simulink model "Longitidunal_Vehicle_Dynamics"  (R2019b)
settings: Solver=VariableStepAuto  StartTime=0.0  StopTime=200  RelTol=1e-3
undefined symbols (not defined in the file): A, a1, a2, cx, g, h, J_w, l, m, mu0, mu1, r, ro, rw, v0
libraries: simulink x1
settings Model: Creator=xps  LastModifiedBy=yanbing_wang
settings SolverCC: ZeroCrossAlgorithm=Adaptive
settings DataIOCC: ReturnWorkspaceOutputs=off
settings DebuggingCC: MaxConsecutiveZCsMsg=none  MaskedZcDiagnostic=none  IgnoredZcDiagnostic=none  ArithmeticOperatorsInVariantConditions=warning
settings SFSimCC: SimUseLocalCustomCode=off  CustomCodeUndefinedFunction=UseInterfaceOnly
settings RTWCC: RTWUseLocalCustomCode=off
settings CodeAppCC: StateflowObjectComments=on

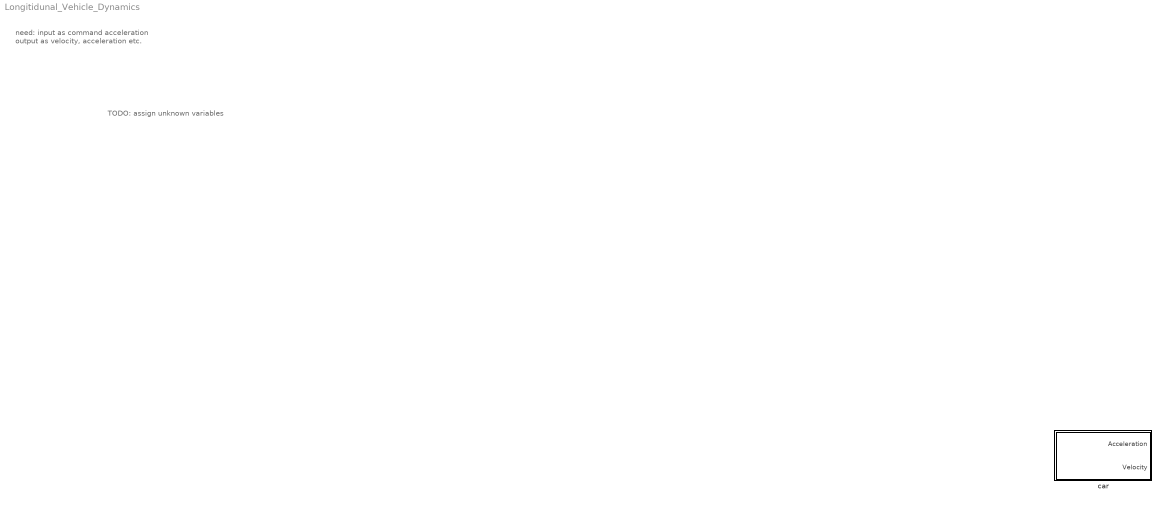
== system Longitidunal_Vehicle_Dynamics ==
  note: TODO: assign unknown variables
  note: need: input as command acceleration
      | output as velocity, acceleration etc.
  car : Subsystem

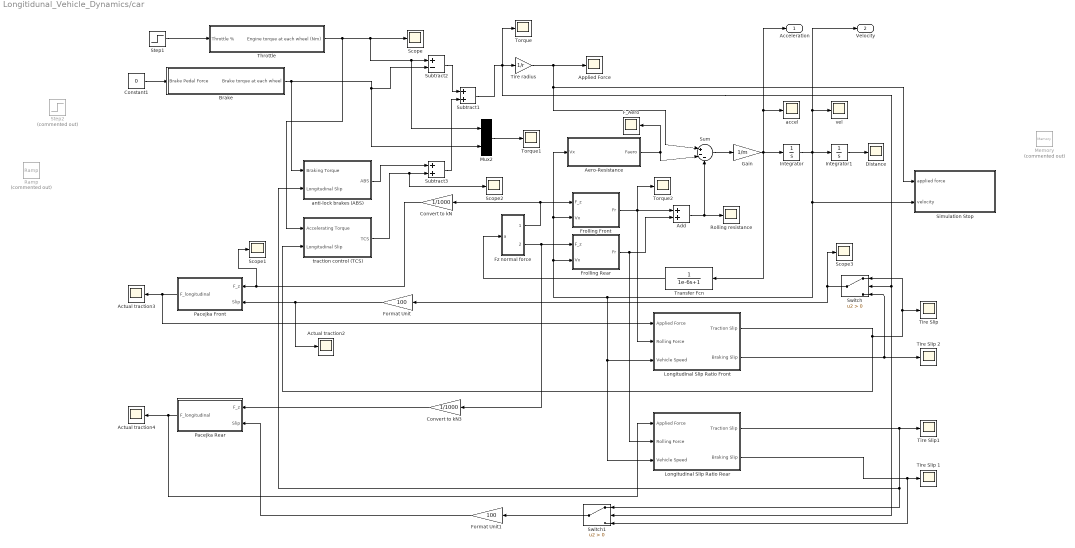
== system Longitidunal_Vehicle_Dynamics/car ==
  Actual traction2 : Scope
  Actual traction3 : Scope
  Actual traction4 : Scope
  Add : Sum
  Aero-Resistance : Subsystem
  Applied Force : Scope
  Brake : Subsystem
  Constant1 : Constant  Value=0
  Convert to kN : Gain  Gain=1/1000
  Convert to kN3 : Gain  Gain=1/1000
  Distance : Scope
  F_Aero : Scope
  Format Unit : Gain  Gain=100
  Format Unit1 : Gain  Gain=100
  Frolling Front : Subsystem
  Frolling Rear : Subsystem
  Fz normal force : Subsystem
  Gain : Gain  Gain=1/m
  Integrator : Integrator  InitialCondition=v0
  Integrator1 : Integrator
  Longitudinal Slip Ratio Front : Subsystem
  Longitudinal Slip Ratio Rear : Subsystem
  Memory : Memory  Commented=on
  Mux2 : Mux  Inputs=2
  Pacejka Front : Subsystem
  Pacejka Rear : Subsystem
  Ramp : simulink/Sources/Ramp  Commented=on  slope=1  start=50  InitialOutput=0
  "Rolling resistance " : Scope
  Scope{,1..3} (4 alike) : Scope
  Simulation Stop : Subsystem
  Step1 : Step  Time=100  After=50  SampleTime=50
  Step2 : Step  Commented=on  Time=100  After=50  SampleTime=1
  Subtract1 : Sum
  Subtract2 : Sum  Inputs=+-
  Subtract3 : Sum
  Sum : Sum  Inputs=|+--
  Switch : Switch  Criteria=u2 > Threshold
  Switch1 : Switch  Criteria=u2 > Threshold
  Throttle : Subsystem
  Tire Slip : Scope
  Tire Slip 1 : Scope
  Tire Slip 2 : Scope
  Tire Slip1 : Scope
  Tire radius : Gain  Gain=1/r
  Torque : Scope
  Torque1 : Scope
  Torque2 : Scope
  Transfer Fcn : TransferFcn  Denominator=[1e-6 1]
  accel : Scope
  anti-lock brakes (ABS) : Subsystem
  traction control (TCS) : Subsystem
  vel : Scope
  Acceleration : Outport
  Velocity : Outport  Port=2
  wires:
  Sum/1 -> Gain/1
  Pacejka Rear/1(F_longitudinal) -> Longitudinal Slip Ratio Rear/1(Applied Force), Actual traction4/1
  Step1/1 -> Throttle/1(Throttle %)
  Format Unit1/1 -> Pacejka Rear/2(Slip)
  Longitudinal Slip Ratio Rear/2(Braking Slip) -> Switch1/3, Tire Slip 1/1
  Integrator1/1 -> Distance/1
  Fz normal force/2(F_z2) -> Convert to kN3/1, Frolling Rear/1(F_z)
  Brake/1(Brake torque at each wheel) -> Subtract2/2, Mux2/2, anti-lock brakes (ABS)/1(Braking Torque)
  Longitudinal Slip Ratio Front/1(Traction Slip) -> traction control (TCS)/2(Longitudinal Slip), Switch/1, Tire Slip/1
  Frolling Rear/1(Fr) -> Longitudinal Slip Ratio Rear/2(Rolling Force), Add/2
  Aero-Resistance/1(Faero) -> Sum/2, F_Aero/1
  Subtract1/1 -> Torque/1, Switch/2, Switch1/2, Tire radius/1
  Subtract2/1 -> Subtract1/1
  Pacejka Front/1(F_longitudinal) -> Actual traction3/1, Longitudinal Slip Ratio Front/1(Applied Force)
  Mux2/1 -> Torque1/1
  traction control (TCS)/1(TCS) -> Scope2/1, Subtract3/2
  Longitudinal Slip Ratio Front/2(Braking Slip) -> Switch/3, Tire Slip 2/1
  Constant1/1 -> Brake/1(Brake Pedal Force)
  Tire radius/1 -> Simulation Stop/1(applied force), Sum/1, Applied Force/1
  Frolling Front/1(Fr) -> Longitudinal Slip Ratio Front/2(Rolling Force), Add/1, Torque2/1
  Longitudinal Slip Ratio Rear/1(Traction Slip) -> anti-lock brakes (ABS)/2(Longitudinal Slip), Switch1/1, Tire Slip1/1
  Subtract3/1 -> Subtract1/2
  anti-lock brakes (ABS)/1(ABS) -> Subtract3/1
  Switch/1 -> Format Unit/1, Scope3/1
  Convert to kN3/1 -> Pacejka Rear/1(F_z)
  Convert to kN/1 -> Scope1/1, Pacejka Front/1(F_z)
  Fz normal force/1(F_z1) -> Convert to kN/1, Frolling Front/1(F_z)
  Switch1/1 -> Format Unit1/1
  Integrator/1 -> Longitudinal Slip Ratio Rear/3(Vehicle Speed), Longitudinal Slip Ratio Front/3(Vehicle Speed), Frolling Front/2(Vx), Aero-Resistance/1(Vx), Frolling Rear/2(Vx), Simulation Stop/2(velocity), Velocity/1, vel/1, Integrator1/1
  Throttle/1(Engine torque at each wheel (Nm)) -> Scope/1, Subtract2/1, Mux2/1, traction control (TCS)/1(Accelerating Torque)
  Add/1 -> Sum/3, "Rolling resistance "/1
  Format Unit/1 -> Pacejka Front/2(Slip), Actual traction2/1
  Gain/1 -> Transfer Fcn/1, Acceleration/1, accel/1, Integrator/1
  Transfer Fcn/1 -> Fz normal force/1(a)

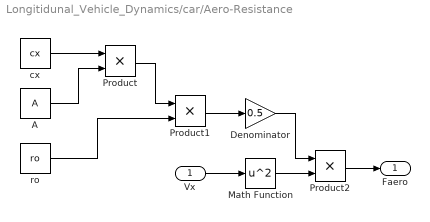
== system Longitidunal_Vehicle_Dynamics/car/Aero-Resistance ==
  Vx : Inport
  A : Constant  Value=A
  Denominator : Gain  Gain=0.5
  Math Function : Math  Operator=square  SaturateOnIntegerOverflow=on
  Product : Product
  Product1 : Product
  Product2 : Product
  cx : Constant  Value=cx
  ro : Constant  Value=ro
  Faero : Outport  VectorParamsAs1DForOutWhenUnconnected=off
  wires:
  A/1 -> Product/2
  Product1/1 -> Denominator/1
  Denominator/1 -> Product2/1
  Vx/1 -> Math Function/1
  Product2/1 -> Faero/1
  ro/1 -> Product1/2
  cx/1 -> Product/1
  Math Function/1 -> Product2/2
  Product/1 -> Product1/1

== system Longitidunal_Vehicle_Dynamics/car/Brake ==
  Brake Pedal Force : Inport
  Gain : Gain  Gain=400
  Gain1 : Gain
  r_static : Gain  Gain=0.3
  Brake torque at each wheel : Outport  VectorParamsAs1DForOutWhenUnconnected=off
  wires:
  Gain1/1 -> r_static/1
  Gain/1 -> Gain1/1
  Brake Pedal Force/1 -> Gain/1
  r_static/1 -> Brake torque at each wheel/1

== system Longitidunal_Vehicle_Dynamics/car/Frolling Front ==
  F_z : Inport
  Vx : Inport  Port=2
  Add : Sum
  Math Function : Math  Operator=square  SaturateOnIntegerOverflow=on
  Product : Product
  Product1 : Product
  mu0 : Constant  Value=mu0
  mu1 : Constant  Value=mu1
  Fr : Outport  VectorParamsAs1DForOutWhenUnconnected=off
  wires:
  Add/1 -> Product1/2
  Math Function/1 -> Product/2
  Product/1 -> Add/2
  mu0/1 -> Add/1
  mu1/1 -> Product/1
  Vx/1 -> Math Function/1
  Product1/1 -> Fr/1
  F_z/1 -> Product1/1

== system Longitidunal_Vehicle_Dynamics/car/Frolling Rear ==
  F_z : Inport
  Vx : Inport  Port=2
  Add : Sum
  Math Function : Math  Operator=square  SaturateOnIntegerOverflow=on
  Product : Product
  Product1 : Product
  mu0 : Constant  Value=mu0
  mu1 : Constant  Value=mu1
  Fr : Outport  VectorParamsAs1DForOutWhenUnconnected=off
  wires:
  F_z/1 -> Product1/1
  Product1/1 -> Fr/1
  Vx/1 -> Math Function/1
  mu1/1 -> Product/1
  mu0/1 -> Add/1
  Product/1 -> Add/2
  Math Function/1 -> Product/2
  Add/1 -> Product1/2

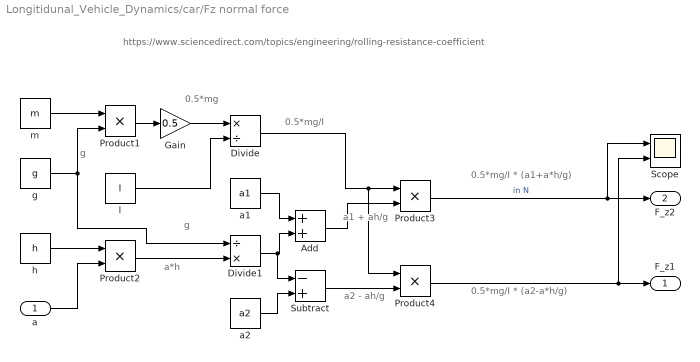
== system Longitidunal_Vehicle_Dynamics/car/Fz normal force ==
  note: https://www.sciencedirect.com/topics/engineering/rolling-resistance-coefficient
  note: a2 - ah/g
  note: a1 + ah/g
  note: 0.5*mg
  note: g
  note: a*h
  note: g
  note: 0.5*mg/I
  note: 0.5*mg/I * (a2-a*h/g)
  note: 0.5*mg/I * (a1+a*h/g)
  a : Inport
  Add : Sum
  Divide : Product  Inputs=*/
  Divide1 : Product  Inputs=/*
  Gain : Gain  Gain=0.5
  Product{1..4} (4 alike) : Product
  Scope : Scope  NumInputPorts=2
  Subtract : Sum  Inputs=-+
  a1 : Constant  Value=a1
  a2 : Constant  Value=a2
  g : Constant  Value=g
  h : Constant  Value=h
  l : Constant  Value=l
  m : Constant  Value=m
  F_z1 : Outport  VectorParamsAs1DForOutWhenUnconnected=off
  F_z2 : Outport  Port=2  VectorParamsAs1DForOutWhenUnconnected=off
  wires:
  m/1 -> Product1/1
  g/1 -> Divide1/1, Product1/2
  Product1/1 -> Gain/1
  Gain/1 -> Divide/1
  l/1 -> Divide/2
  h/1 -> Product2/1
  Product2/1 -> Divide1/2
  a1/1 -> Add/1
  Divide1/1 -> Subtract/1, Add/2
  Divide/1 -> Product4/1, Product3/1
  Add/1 -> Product3/2
  a2/1 -> Subtract/2
  Subtract/1 -> Product4/2
  Product4/1 -> Scope/2, F_z1/1
  Product3/1 -> Scope/1, F_z2/1  "in N"
  a/1 -> Product2/2

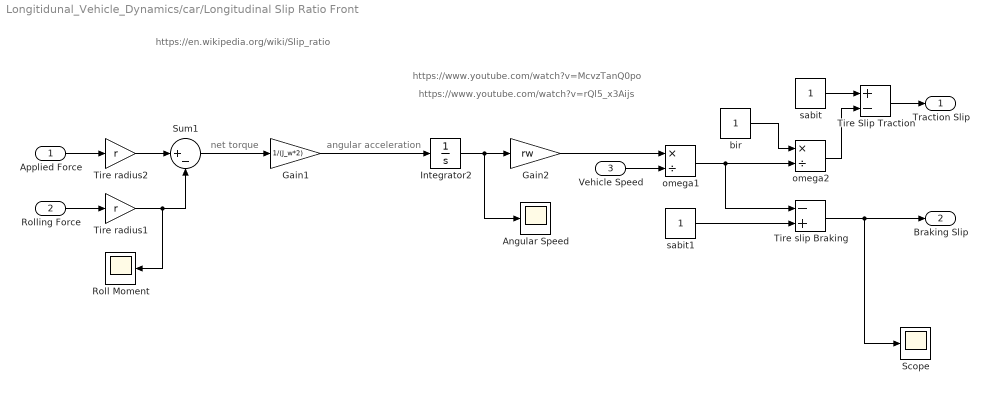
== system Longitidunal_Vehicle_Dynamics/car/Longitudinal Slip Ratio Front ==
  note: https://www.youtube.com/watch?v=McvzTanQ0po
  note: net torque
  note: https://www.youtube.com/watch?v=rQl5_x3Aijs
  note: angular acceleration
  note: https://en.wikipedia.org/wiki/Slip_ratio
  Applied Force : Inport
  Rolling Force : Inport  Port=2
  Vehicle Speed : Inport  Port=3
  Angular Speed : Scope
  Gain1 : Gain  Gain=1/(J_w*2)
  Gain2 : Gain  Gain=rw
  Integrator2 : Integrator  InitialCondition=0.00001
  Roll Moment : Scope
  Scope : Scope
  Sum1 : Sum  Inputs=|+-
  Tire Slip Traction : Sum  Inputs=+-
  Tire radius1 : Gain  Gain=r
  Tire radius2 : Gain  Gain=r
  Tire slip Braking : Sum  Inputs=-+
  bir : Constant
  omega1 : Product  Inputs=*/
  omega2 : Product  Inputs=*/
  sabit : Constant
  sabit1 : Constant
  Traction Slip : Outport  VectorParamsAs1DForOutWhenUnconnected=off
  Braking Slip : Outport  Port=2  VectorParamsAs1DForOutWhenUnconnected=off
  wires:
  Rolling Force/1 -> Tire radius1/1
  Vehicle Speed/1 -> omega1/2
  Tire slip Braking/1 -> Scope/1, Braking Slip/1
  Integrator2/1 -> Gain2/1, Angular Speed/1
  sabit/1 -> Tire Slip Traction/1
  bir/1 -> omega2/1
  omega2/1 -> Tire Slip Traction/2
  Tire Slip Traction/1 -> Traction Slip/1
  Gain1/1 -> Integrator2/1
  Gain2/1 -> omega1/1
  omega1/1 -> Tire slip Braking/1, omega2/2
  Tire radius1/1 -> Sum1/2, Roll Moment/1
  sabit1/1 -> Tire slip Braking/2
  Applied Force/1 -> Tire radius2/1
  Sum1/1 -> Gain1/1
  Tire radius2/1 -> Sum1/1

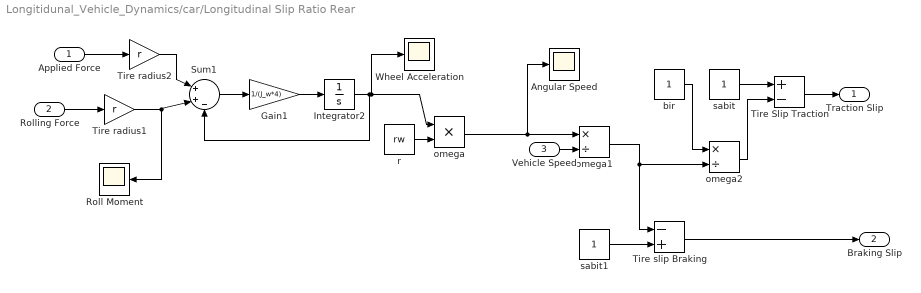
== system Longitidunal_Vehicle_Dynamics/car/Longitudinal Slip Ratio Rear ==
  Applied Force : Inport
  Rolling Force : Inport  Port=2
  Vehicle Speed : Inport  Port=3
  Angular Speed : Scope
  Gain1 : Gain  Gain=1/(J_w*4)
  Integrator2 : Integrator  InitialCondition=0.00001
  Roll Moment : Scope
  Sum1 : Sum  Inputs=|++-
  Tire Slip Traction : Sum  Inputs=+-
  Tire radius1 : Gain  Gain=r
  Tire radius2 : Gain  Gain=r
  Tire slip Braking : Sum  Inputs=-+
  Wheel Acceleration : Scope
  bir : Constant
  omega : Product  Inputs=**
  omega1 : Product  Inputs=*/
  omega2 : Product  Inputs=*/
  r : Constant  Value=rw
  sabit : Constant
  sabit1 : Constant
  Traction Slip : Outport  VectorParamsAs1DForOutWhenUnconnected=off
  Braking Slip : Outport  Port=2  VectorParamsAs1DForOutWhenUnconnected=off
  wires:
  sabit1/1 -> Tire slip Braking/2
  Tire radius1/1 -> Roll Moment/1, Sum1/2
  omega1/1 -> omega2/2, Tire slip Braking/1
  omega/1 -> omega1/1, Angular Speed/1
  r/1 -> omega/2
  Gain1/1 -> Integrator2/1
  Tire Slip Traction/1 -> Traction Slip/1
  omega2/1 -> Tire Slip Traction/2
  bir/1 -> omega2/1
  Sum1/1 -> Gain1/1
  sabit/1 -> Tire Slip Traction/1
  Integrator2/1 -> Wheel Acceleration/1, omega/1, Sum1/3
  Tire slip Braking/1 -> Braking Slip/1
  Vehicle Speed/1 -> omega1/2
  Applied Force/1 -> Tire radius2/1
  Rolling Force/1 -> Tire radius1/1
  Tire radius2/1 -> Sum1/1

== system Longitidunal_Vehicle_Dynamics/car/Pacejka Front ==
  F_z : Inport
  Slip : Inport  Port=2
  Longitudinal : Subsystem
  Subsystem : Subsystem
  F_longitudinal : Outport  VectorParamsAs1DForOutWhenUnconnected=off
  wires:
  Longitudinal/1(F) -> F_longitudinal/1
  F_z/1 -> Subsystem/1(F_z)
  Slip/1 -> Subsystem/2(slip)
  Subsystem/4(E) -> Longitudinal/3(E)
  Subsystem/5(Bx1) -> Longitudinal/4(Bx1)
  Subsystem/1(C) -> Longitudinal/1(C)
  Subsystem/2(D) -> Longitudinal/2(D)
  Subsystem/3(V) -> Longitudinal/5(V)

== system Longitidunal_Vehicle_Dynamics/car/Pacejka Rear ==
  F_z : Inport
  Slip : Inport  Port=2
  Longitudinal : Subsystem
  Subsystem : Subsystem
  F_longitudinal : Outport  VectorParamsAs1DForOutWhenUnconnected=off
  wires:
  Longitudinal/1(F) -> F_longitudinal/1
  F_z/1 -> Subsystem/1(F_z)
  Slip/1 -> Subsystem/2(slip)
  Subsystem/4(E) -> Longitudinal/3(E)
  Subsystem/5(Bx1) -> Longitudinal/4(Bx1)
  Subsystem/1(C) -> Longitudinal/1(C)
  Subsystem/2(D) -> Longitudinal/2(D)
  Subsystem/3(V) -> Longitudinal/5(V)

== system Longitidunal_Vehicle_Dynamics/car/Simulation Stop ==
  applied force : Inport
  velocity : Inport  Port=2
  Constant : Constant  Value=0.01
  Constant1 : Constant  Value=0
  Logical Operator : Logic  Operator=OR  AllPortsSameDT=off  OutDataTypeStr=boolean
  Relational Operator : RelationalOperator  Operator=<=  OutDataTypeStr=boolean  RndMeth=Simplest
  Relational Operator1 : RelationalOperator  Operator=<  OutDataTypeStr=boolean  RndMeth=Simplest
  Stop Simulation : Stop
  wires:
  Constant/1 -> Relational Operator/2
  velocity/1 -> Relational Operator/1
  Relational Operator1/1 -> Logical Operator/1
  Constant1/1 -> Relational Operator1/2
  applied force/1 -> Relational Operator1/1
  Logical Operator/1 -> Stop Simulation/1
  Relational Operator/1 -> Logical Operator/2

== system Longitidunal_Vehicle_Dynamics/car/Throttle ==
  Throttle % : Inport
  Gain : Gain  Gain=2.4
  Gain1 : Gain
  Engine torque at each wheel (Nm) : Outport  VectorParamsAs1DForOutWhenUnconnected=off
  wires:
  Gain/1 -> Gain1/1
  Throttle %/1 -> Gain/1
  Gain1/1 -> Engine torque at each wheel (Nm)/1

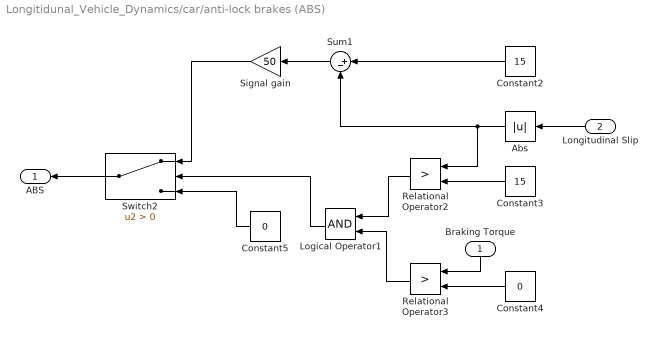
== system Longitidunal_Vehicle_Dynamics/car/anti-lock brakes (ABS) ==
  Braking Torque : Inport
  Longitudinal Slip : Inport  Port=2
  Abs : Abs
  Constant2 : Constant  Value=15
  Constant3 : Constant  Value=15
  Constant4 : Constant  Value=0
  Constant5 : Constant  Value=0
  Logical Operator1 : Logic  AllPortsSameDT=off  OutDataTypeStr=boolean
  Relational Operator2 : RelationalOperator  Operator=>  OutDataTypeStr=boolean  RndMeth=Simplest
  Relational Operator3 : RelationalOperator  Operator=>  OutDataTypeStr=boolean  RndMeth=Simplest
  Signal gain : Gain  Gain=50
  Sum1 : Sum  Inputs=|+-
  Switch2 : Switch  Criteria=u2 > Threshold
  ABS : Outport  VectorParamsAs1DForOutWhenUnconnected=off
  wires:
  Sum1/1 -> Signal gain/1
  Constant4/1 -> Relational Operator3/2
  Longitudinal Slip/1 -> Abs/1
  Braking Torque/1 -> Relational Operator3/1
  Switch2/1 -> ABS/1
  Relational Operator2/1 -> Logical Operator1/1
  Constant3/1 -> Relational Operator2/2
  Logical Operator1/1 -> Switch2/2
  Constant2/1 -> Sum1/1
  Relational Operator3/1 -> Logical Operator1/2
  Constant5/1 -> Switch2/3
  Abs/1 -> Relational Operator2/1, Sum1/2
  Signal gain/1 -> Switch2/1

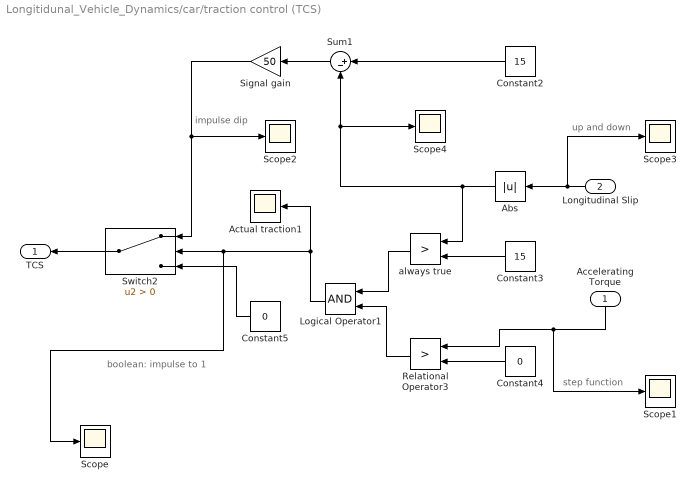
== system Longitidunal_Vehicle_Dynamics/car/traction control (TCS) ==
  note: step function
  note: up and down
  note: impulse dip
  note: boolean: impulse to 1
  Accelerating Torque : Inport
  Longitudinal Slip : Inport  Port=2
  Abs : Abs
  Actual traction1 : Scope
  Constant2 : Constant  Value=15
  Constant3 : Constant  Value=15
  Constant4 : Constant  Value=0
  Constant5 : Constant  Value=0
  Logical Operator1 : Logic  AllPortsSameDT=off  OutDataTypeStr=boolean
  Relational Operator3 : RelationalOperator  Operator=>  OutDataTypeStr=boolean  RndMeth=Simplest
  Scope{,1..4} (5 alike) : Scope
  Signal gain : Gain  Gain=50
  Sum1 : Sum  Inputs=|+-
  Switch2 : Switch  Criteria=u2 > Threshold
  always true : RelationalOperator  Operator=>  OutDataTypeStr=boolean  RndMeth=Simplest
  TCS : Outport  VectorParamsAs1DForOutWhenUnconnected=off
  wires:
  Signal gain/1 -> Scope2/1, Switch2/1
  Longitudinal Slip/1 -> Abs/1, Scope3/1
  Constant5/1 -> Switch2/3
  Relational Operator3/1 -> Logical Operator1/2
  Constant2/1 -> Sum1/1
  Logical Operator1/1 -> Actual traction1/1, Scope/1, Switch2/2
  Constant3/1 -> always true/2
  always true/1 -> Logical Operator1/1
  Switch2/1 -> TCS/1
  Accelerating Torque/1 -> Scope1/1, Relational Operator3/1
  Constant4/1 -> Relational Operator3/2
  Sum1/1 -> Signal gain/1
  Abs/1 -> Scope4/1, Sum1/2, always true/1

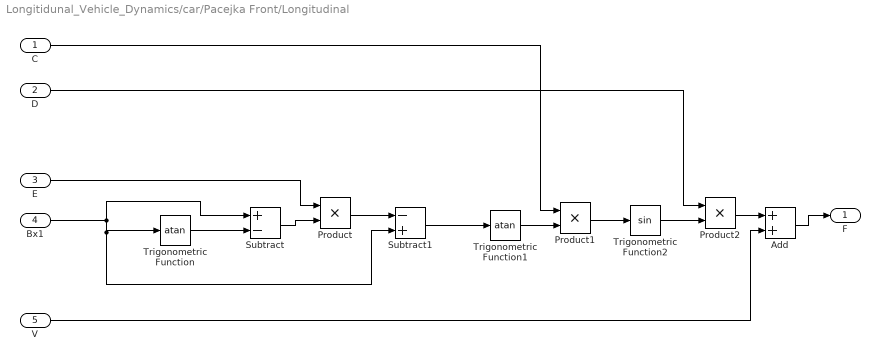
== system Longitidunal_Vehicle_Dynamics/car/Pacejka Front/Longitudinal ==
  C : Inport
  D : Inport  Port=2
  E : Inport  Port=3
  Bx1 : Inport  Port=4
  V : Inport  Port=5
  Add : Sum
  Product : Product
  Product1 : Product
  Product2 : Product
  Subtract : Sum  Inputs=+-
  Subtract1 : Sum  Inputs=-+
  Trigonometric Function : Trigonometry  Operator=atan
  Trigonometric Function1 : Trigonometry  Operator=atan
  Trigonometric Function2 : Trigonometry
  F : Outport  VectorParamsAs1DForOutWhenUnconnected=off
  wires:
  Subtract/1 -> Product/2
  Trigonometric Function/1 -> Subtract/2
  Product/1 -> Subtract1/1
  Trigonometric Function1/1 -> Product1/2
  D/1 -> Product2/1
  Product1/1 -> Trigonometric Function2/1
  Trigonometric Function2/1 -> Product2/2
  Bx1/1 -> Trigonometric Function/1, Subtract1/2, Subtract/1
  Subtract1/1 -> Trigonometric Function1/1
  E/1 -> Product/1
  C/1 -> Product1/1
  Product2/1 -> Add/1
  V/1 -> Add/2
  Add/1 -> F/1

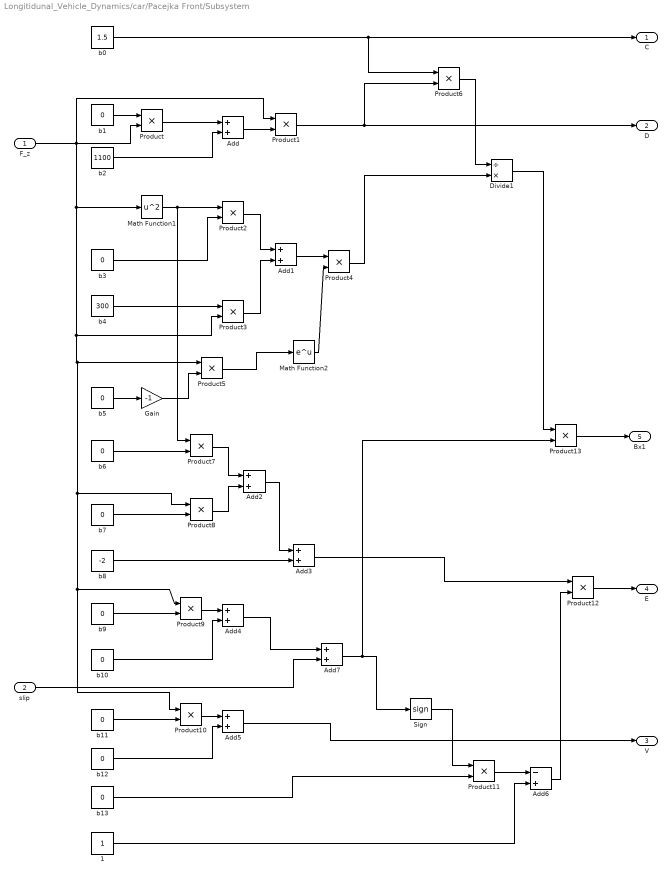
== system Longitidunal_Vehicle_Dynamics/car/Pacejka Front/Subsystem ==
  F_z : Inport
  slip : Inport  Port=2
  1 : Constant
  Add{,1..5,7} (7 alike) : Sum
  Add6 : Sum  Inputs=-+
  Divide1 : Product  Inputs=/*
  Gain : Gain  Gain=-1
  Math Function1 : Math  Operator=square  SaturateOnIntegerOverflow=on
  Math Function2 : Math  SaturateOnIntegerOverflow=on
  Product{,1..13} (14 alike) : Product
  Sign : Signum
  b0 : Constant  Value=1.5
  b{1,3,5..7,9..13} (10 alike) : Constant  Value=0
  b2 : Constant  Value=1100
  b4 : Constant  Value=300
  b8 : Constant  Value=-2
  C : Outport  VectorParamsAs1DForOutWhenUnconnected=off
  D : Outport  Port=2  VectorParamsAs1DForOutWhenUnconnected=off
  V : Outport  Port=3  VectorParamsAs1DForOutWhenUnconnected=off
  E : Outport  Port=4  VectorParamsAs1DForOutWhenUnconnected=off
  Bx1 : Outport  Port=5  VectorParamsAs1DForOutWhenUnconnected=off
  wires:
  Add3/1 -> Product12/1
  Add1/1 -> Product4/1
  1/1 -> Add6/2
  b13/1 -> Product11/2
  slip/1 -> Add7/2
  Product12/1 -> E/1
  Product2/1 -> Add1/1
  Sign/1 -> Product11/1
  Add7/1 -> Product13/2, Sign/1
  Math Function2/1 -> Product4/2
  b6/1 -> Product7/2
  Product13/1 -> Bx1/1
  Product11/1 -> Add6/1
  b12/1 -> Add5/2
  b10/1 -> Add4/2
  b8/1 -> Add3/2
  b7/1 -> Product8/2
  Add6/1 -> Product12/2
  Product9/1 -> Add4/1
  Product4/1 -> Divide1/2
  Math Function1/1 -> Product7/1, Product2/1
  b0/1 -> C/1, Product6/1
  b2/1 -> Add/2
  Add5/1 -> V/1
  b9/1 -> Product9/2
  b1/1 -> Product/1
  F_z/1 -> Product3/2, Product10/1, Product9/1, Product8/1, Product5/1, Math Function1/1, Product1/1, Product/2
  Product/1 -> Add/1
  Gain/1 -> Product5/2
  Divide1/1 -> Product13/1
  b4/1 -> Product3/1
  Add/1 -> Product1/2
  Add4/1 -> Add7/1
  Product10/1 -> Add5/1
  Product5/1 -> Math Function2/1
  Add2/1 -> Add3/1
  Product6/1 -> Divide1/1
  b5/1 -> Gain/1
  Product8/1 -> Add2/2
  Product7/1 -> Add2/1
  Product3/1 -> Add1/2
  b3/1 -> Product2/2
  b11/1 -> Product10/2
  Product1/1 -> D/1, Product6/2

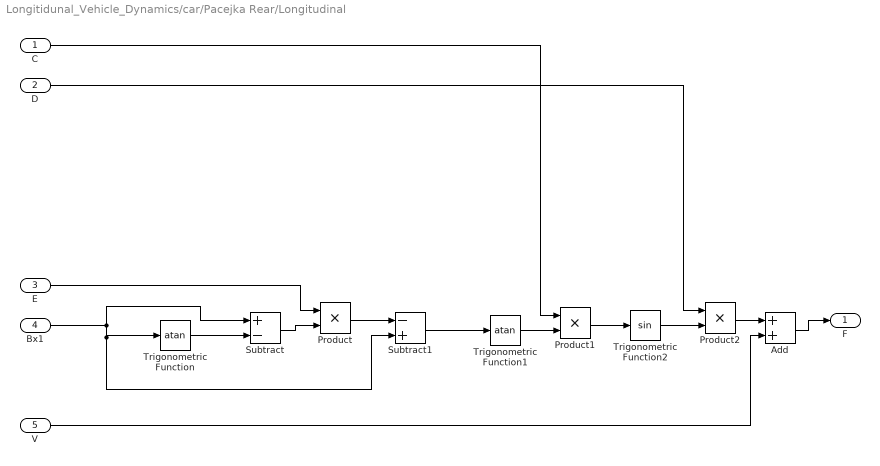
== system Longitidunal_Vehicle_Dynamics/car/Pacejka Rear/Longitudinal ==
  C : Inport
  D : Inport  Port=2
  E : Inport  Port=3
  Bx1 : Inport  Port=4
  V : Inport  Port=5
  Add : Sum
  Product : Product
  Product1 : Product
  Product2 : Product
  Subtract : Sum  Inputs=+-
  Subtract1 : Sum  Inputs=-+
  Trigonometric Function : Trigonometry  Operator=atan
  Trigonometric Function1 : Trigonometry  Operator=atan
  Trigonometric Function2 : Trigonometry
  F : Outport  VectorParamsAs1DForOutWhenUnconnected=off
  wires:
  Subtract/1 -> Product/2
  Trigonometric Function/1 -> Subtract/2
  Product/1 -> Subtract1/1
  Trigonometric Function1/1 -> Product1/2
  D/1 -> Product2/1
  Product1/1 -> Trigonometric Function2/1
  Trigonometric Function2/1 -> Product2/2
  Bx1/1 -> Trigonometric Function/1, Subtract1/2, Subtract/1
  Subtract1/1 -> Trigonometric Function1/1
  E/1 -> Product/1
  C/1 -> Product1/1
  Product2/1 -> Add/1
  V/1 -> Add/2
  Add/1 -> F/1

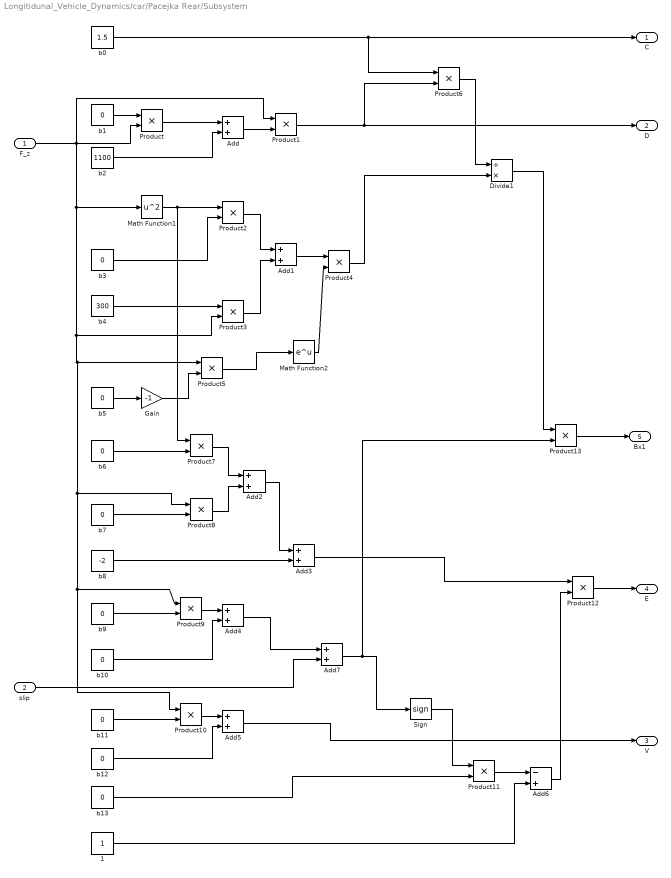
== system Longitidunal_Vehicle_Dynamics/car/Pacejka Rear/Subsystem ==
  F_z : Inport
  slip : Inport  Port=2
  1 : Constant
  Add{,1..5,7} (7 alike) : Sum
  Add6 : Sum  Inputs=-+
  Divide1 : Product  Inputs=/*
  Gain : Gain  Gain=-1
  Math Function1 : Math  Operator=square  SaturateOnIntegerOverflow=on
  Math Function2 : Math  SaturateOnIntegerOverflow=on
  Product{,1..13} (14 alike) : Product
  Sign : Signum
  b0 : Constant  Value=1.5
  b{1,3,5..7,9..13} (10 alike) : Constant  Value=0
  b2 : Constant  Value=1100
  b4 : Constant  Value=300
  b8 : Constant  Value=-2
  C : Outport  VectorParamsAs1DForOutWhenUnconnected=off
  D : Outport  Port=2  VectorParamsAs1DForOutWhenUnconnected=off
  V : Outport  Port=3  VectorParamsAs1DForOutWhenUnconnected=off
  E : Outport  Port=4  VectorParamsAs1DForOutWhenUnconnected=off
  Bx1 : Outport  Port=5  VectorParamsAs1DForOutWhenUnconnected=off
  wires:
  Add3/1 -> Product12/1
  Add1/1 -> Product4/1
  1/1 -> Add6/2
  b13/1 -> Product11/2
  slip/1 -> Add7/2
  Product12/1 -> E/1
  Product2/1 -> Add1/1
  Sign/1 -> Product11/1
  Add7/1 -> Product13/2, Sign/1
  Math Function2/1 -> Product4/2
  b6/1 -> Product7/2
  Product13/1 -> Bx1/1
  Product11/1 -> Add6/1
  b12/1 -> Add5/2
  b10/1 -> Add4/2
  b8/1 -> Add3/2
  b7/1 -> Product8/2
  Add6/1 -> Product12/2
  Product9/1 -> Add4/1
  Product4/1 -> Divide1/2
  Math Function1/1 -> Product7/1, Product2/1
  b0/1 -> C/1, Product6/1
  b2/1 -> Add/2
  Add5/1 -> V/1
  b9/1 -> Product9/2
  b1/1 -> Product/1
  F_z/1 -> Product3/2, Product10/1, Product9/1, Product8/1, Product5/1, Math Function1/1, Product1/1, Product/2
  Product/1 -> Add/1
  Gain/1 -> Product5/2
  Divide1/1 -> Product13/1
  b4/1 -> Product3/1
  Add/1 -> Product1/2
  Add4/1 -> Add7/1
  Product10/1 -> Add5/1
  Product5/1 -> Math Function2/1
  Add2/1 -> Add3/1
  Product6/1 -> Divide1/1
  b5/1 -> Gain/1
  Product8/1 -> Add2/2
  Product7/1 -> Add2/1
  Product3/1 -> Add1/2
  b3/1 -> Product2/2
  b11/1 -> Product10/2
  Product1/1 -> D/1, Product6/2
